simulink model "identyfikacja_zawor1_reczny"  (R2014b)
settings: Solver=ode5  StartTime=0.0  StopTime=40.45  FixedStep=0.05  RelTol=1e-3
values from neighbouring files (symbols this model uses):
  a = 31    [charakterystyka_pompa.m]    (also in charakterystyka_pompa_sterownik.m; dane14listopad.mat; danePompa.mat; pomiary.m)
  C1 = q/sqrt(H1pp)    [linearyzacja_analitycznie.m]    (also in wskaznikZawor1.m = parametry(1))
  w = 5    [charakterystyka_pompa.m]    (also in charakterystyka_pompa_sterownik.m; dane14listopad.mat; danePompa.mat; pomiary.m)
  x01 = 33    [identyfikacja_zawor1.m]    (also in wskaznikZawor1.m = parametry(2))
settings Model: Creator=Michal  LastModifiedBy=Michal
settings DebuggingCC: UnderspecifiedInitializationDetection=Classic  MergeDetectMultiDrivingBlocksExec=none

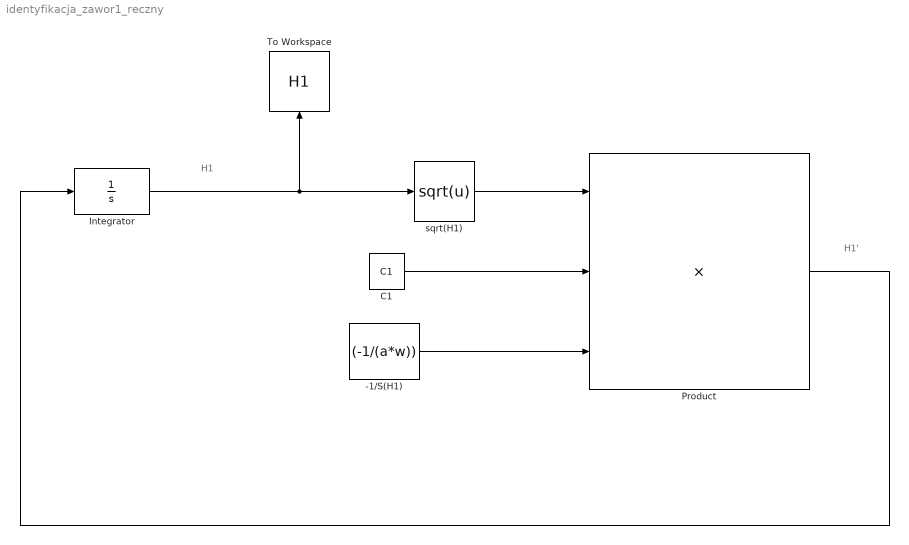
== system identyfikacja_zawor1_reczny ==
  note: H1'
  note: H1
  -1/S(H1) : Constant  Value=(-1/(a*w))
  "C1 " : Constant  Value=C1
  Integrator : Integrator  InitialCondition=x01
  Product : Product  Inputs=3
  To Workspace : ToWorkspace  VariableName=H1  SaveFormat=Structure With Time  SampleTime=-1
  sqrt(H1) : Fcn  Expr=sqrt(u)
  wires:
  "C1 "/1 -> Product/2
  Product/1 -> Integrator/1
  -1/S(H1)/1 -> Product/3
  sqrt(H1)/1 -> Product/1
  Integrator/1 -> sqrt(H1)/1, To Workspace/1
